simulink model "MLC_Aero_model"  (R2017a)
settings: Solver=VariableStepAuto  StartTime=0.0  StopTime=100  RelTol=1e-3
libraries: cstblocks x6
settings Model: Creator=harsh  LastModifiedBy=harsh

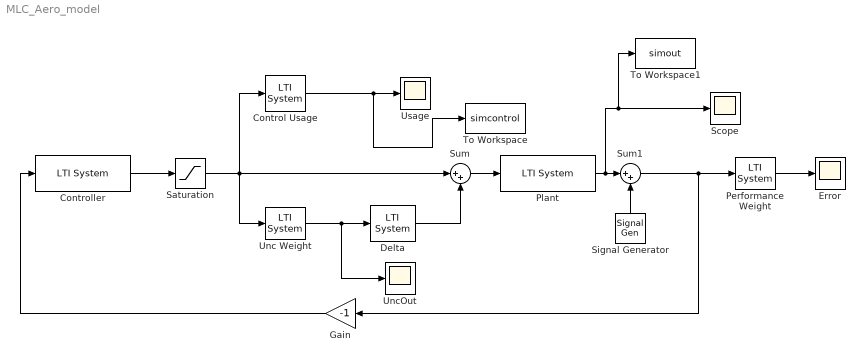
== system MLC_Aero_model ==
  Control Usage : cstblocks/LTI System  sys=Wu  IC=[]
  Controller : cstblocks/LTI System  sys=K  IC=[]
  "Delta " : cstblocks/LTI System  sys=Del_I  IC=[]
  Error : Scope
  Gain : Gain  Gain=-1
  Performance Weight : cstblocks/LTI System  sys=Wp  IC=[]
  Plant : cstblocks/LTI System  sys=Gnom  IC=[]
  Saturation : Saturate  UpperLimit=25  LowerLimit=-25
  Scope : Scope
  Signal Generator : SignalGenerator  WaveForm=square  Amplitude=[pi/4;pi/6]  Frequency=[0.5;0.4]  Units=rad/sec
  Sum : Sum  Inputs=|++
  Sum1 : Sum  Inputs=|++
  To Workspace : ToWorkspace  VariableName=simcontrol  SaveFormat=Structure With Time  SampleTime=-1
  To Workspace1 : ToWorkspace  VariableName=simout  SaveFormat=Structure With Time  SampleTime=-1
  Unc Weight : cstblocks/LTI System  sys=WI  IC=[]
  UncOut : Scope
  "Usage " : Scope
  wires:
  Controller/1 -> Saturation/1
  Sum/1 -> Plant/1
  Saturation/1 -> Control Usage/1, Unc Weight/1, Sum/1
  Unc Weight/1 -> UncOut/1, "Delta "/1
  "Delta "/1 -> Sum/2
  Control Usage/1 -> To Workspace/1, "Usage "/1
  Plant/1 -> To Workspace1/1, Scope/1, Sum1/1
  Performance Weight/1 -> Error/1
  Signal Generator/1 -> Sum1/2
  Sum1/1 -> Gain/1, Performance Weight/1
  Gain/1 -> Controller/1
